simulink model "lab1_3"  (R2026a)
settings: Solver=VariableStepAuto  StopTime=inf
undefined symbols (not defined in the file): Blocking, Non
libraries: amg_usbconverter_n_connect_lib x2
settings Model: Creator=Asus  LastModifiedBy=Asus

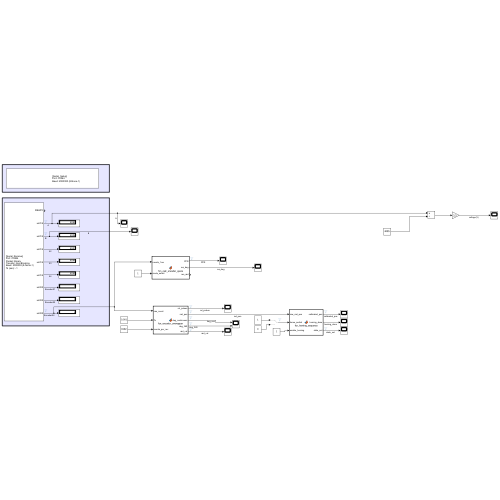
[thumbnail: Simulink's stored preview of the top-level diagram]
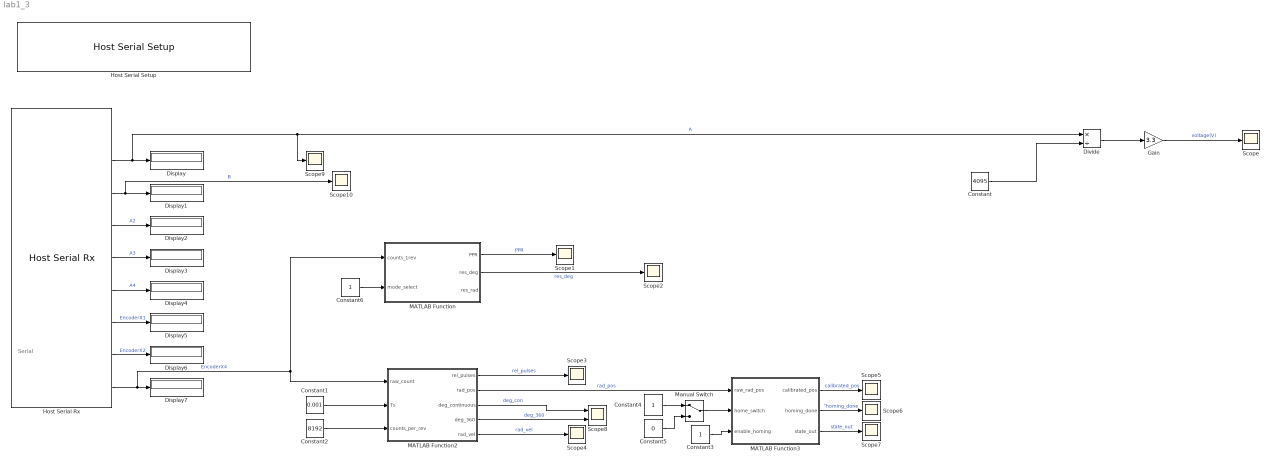
== system lab1_3 ==
  note: Serial
  Constant : Constant  Value=4095
  Constant1 : Constant  Value=0.001
  Constant2 : Constant  Value=8192
  Constant3 : Constant
  Constant4 : Constant  OutDataTypeStr=boolean
  Constant5 : Constant  Value=0  OutDataTypeStr=boolean
  Constant6 : Constant
  Display{,1..7} (8 alike) : Display
  Divide : Product  Inputs=*/
  Gain : Gain  Gain=3.3
  Host Serial Rx : amg_usbconverter_n_connect_lib/Host Serial Rx  conf=rx  port=<auto>  baudrate=2000000  databits=8  parity=None  stopbit=1  flowcontrol=None  transfer=Non-Blocking  timeout=5  packetmode=Binary  enableinitialvalues=off  initialvalues=[]  binheader='25'  binterminator='4E 4E'  porttype_double=0  porttype_single=0  porttype_int8=0  porttype_uint8=0  porttype_int16=0  porttype_uint16=5  porttype_int32=0  porttype_uint32=3  asciiformat='%d,%f'  rx_asciiterminator="CRLF (0x0D 0x0A - \"\\r\\n\")"  tx_asciiterminator="CRLF (0x0D 0x0A - \"\\r\\n\")"  sampletime=0.001  enablecustomportlabel=off  cinputportlabel=0  coutputportlabel=A  portpinstr=0  blockid=HostSerialRx  inputporttype=[]  inputportwidth=[]  inputportlabel={}  outputporttype=[3 5 5 5 5 5 7 7 7]  outputportwidth=[1 1 1 1 1 1 1 1 1]  outputportlabel={'READY','uint16','uint16','uint16','uint16','uint16','uint32','uint32','uint32'}  compat=0  optionstring=[]  autoport='COM4'
  Host Serial Setup : amg_usbconverter_n_connect_lib/Host Serial Setup  conf=setup  port=<auto>  baudrate=2000000  databits=8  parity=None  stopbit=1  flowcontrol=None  transfer=Blocking  timeout=2  packetmode=Binary  initialvalues=[]  binheader='7E 7E'  binterminator='03 03'  porttype_double=0  porttype_single=1  porttype_int8=0  porttype_uint8=0  porttype_int16=0  porttype_uint16=0  porttype_int32=0  porttype_uint32=2  asciiformat='%d %u %x'  rx_asciiterminator="CRLF (0x0D 0x0A - \"\\r\\n\")"  tx_asciiterminator="CRLF (0x0D 0x0A - \"\\r\\n\")"  sampletime=-1  enablecustomportlabel=off  cinputportlabel=0  coutputportlabel=A  portpinstr=0  blockid=HostSerialSetup  inputporttype=[]  inputportwidth=[]  inputportlabel={}  outputporttype=[]  outputportwidth=[]  outputportlabel={}  compat=0  optionstring=[]  autoport='COM4'
  MATLAB Function : MATLAB Function  TreatAsAtomicUnit=on
  MATLAB Function2 : MATLAB Function  TreatAsAtomicUnit=on
  MATLAB Function3 : MATLAB Function  TreatAsAtomicUnit=on
  Manual Switch : ManualSwitch
  Scope{,1..7,9..10} (10 alike) : Scope
      Scope settings: ActiveDisplayYMinimum=-29.471685212947058  ActiveDisplayYMaximum=19.265337201699708
      Scope1 settings: ActiveDisplayYMinimum=-29.471685212947058  ActiveDisplayYMaximum=19.265337201699708
      Scope10 settings: DataLoggingVariableName=ScopeData10
      Scope2 settings: ActiveDisplayYMinimum=-29.471685212947058  ActiveDisplayYMaximum=19.265337201699708  DataLoggingVariableName=ScopeData2
      Scope3 settings: ActiveDisplayYMinimum=-29.471685212947058  ActiveDisplayYMaximum=19.265337201699708  DataLoggingVariableName=ScopeData3
      Scope4 settings: ActiveDisplayYMinimum=-29.471685212947058  ActiveDisplayYMaximum=19.265337201699708  DataLoggingVariableName=ScopeData4
      Scope5 settings: ActiveDisplayYMinimum=-29.471685212947058  ActiveDisplayYMaximum=19.265337201699708  DataLoggingVariableName=ScopeData5
      Scope6 settings: ActiveDisplayYMinimum=-29.471685212947058  ActiveDisplayYMaximum=19.265337201699708  DataLoggingVariableName=ScopeData6
      Scope7 settings: ActiveDisplayYMinimum=-29.471685212947058  ActiveDisplayYMaximum=19.265337201699708  DataLoggingVariableName=ScopeData7
      Scope9 settings: DataLoggingVariableName=ScopeData9
  Scope8 : Scope  NumInputPorts=2
      settings: ActiveDisplayYMinimum=-29.471685212947058  ActiveDisplayYMaximum=19.265337201699708  DataLoggingVariableName=ScopeData8
  wires:
  Host Serial Rx/6 -> Display4/1  "A4"
  Host Serial Rx/9 -> MATLAB Function2/1(raw_count), MATLAB Function/1(counts_1rev), Display7/1  "EncoderX4"
  Constant/1 -> Divide/2
  Host Serial Rx/7 -> Display5/1  "EncoderX1"
  Divide/1 -> Gain/1
  Host Serial Rx/8 -> Display6/1  "EncoderX2"
  Host Serial Rx/3 -> Scope10/1, Display1/1  "B"
  Host Serial Rx/5 -> Display3/1  "A3"
  Host Serial Rx/2 -> Scope9/1, Divide/1, Display/1  "A"
  Gain/1 -> Scope/1  "voltage(V)"
  Host Serial Rx/4 -> Display2/1  "A2"
  Constant1/1 -> MATLAB Function2/2(Ts)
  Constant2/1 -> MATLAB Function2/3(counts_per_rev)
  MATLAB Function2/2(rad_pos) -> MATLAB Function3/1(raw_rad_pos)  "rad_pos"
  Constant3/1 -> MATLAB Function3/3(enable_homing)
  Manual Switch/1 -> MATLAB Function3/2(home_switch)
  Constant4/1 -> Manual Switch/1
  Constant5/1 -> Manual Switch/2
  Constant6/1 -> MATLAB Function/2(mode_select)
  MATLAB Function/1(PPR) -> Scope1/1  "PPR"
  MATLAB Function/2(res_deg) -> Scope2/1  "res_deg"
  MATLAB Function2/5(rad_vel) -> Scope4/1  "rad_vel"
  MATLAB Function2/1(rel_pulses) -> Scope3/1  "rel_pulses"
  MATLAB Function3/1(calibrated_pos) -> Scope5/1  "calibrated_pos"
  MATLAB Function3/2(homing_done) -> Scope6/1  "้homing_done"
  MATLAB Function3/3(state_out) -> Scope7/1  "state_out"
  MATLAB Function2/3(deg_continuous) -> Scope8/1  "deg_con"
  MATLAB Function2/4(deg_360) -> Scope8/2  "deg_360"

== matlab function lab1_3/MATLAB Function ==
  data: counts_1rev input; PPR output; mode_select input; res_deg output; res_rad output
function [PPR, res_deg, res_rad] = fcn_calc_encoder_specs(counts_1rev, mode_select)
% FCN_CALC_ENCODER_SPECS
% คำนวณ PPR และ Angular Resolution (แปลง Type เป็น double ป้องกัน Type Mismatch)

% 1. บังคับแปลง Input ทุกตัวเป็น double ป้องกันการตัดเศษทศนิยมและ Data Type ขัดแย้ง
c = double(counts_1rev);
m = double(mode_select);

% 2. คำนวณค่าตามเงื่อนไข
if c > 0 && m > 0
    PPR     = c / m;
    res_deg = 360.0 / c;
    res_rad = (2.0 * pi) / c;
else
    PPR     = 0.0;
    res_deg = 0.0;
    res_rad = 0.0;
end
end

== matlab function lab1_3/MATLAB Function2 ==
  data: raw_count input; rel_pulses output; Ts input; counts_per_rev input; rad_pos output; deg_continuous output; deg_360 output; rad_vel output
function [rel_pulses, rad_pos, deg_continuous, deg_360, rad_vel] = fcn_encoder_unwrapper(raw_count, Ts, counts_per_rev)
    persistent prev_raw accumulated_pulses prev_rad_pos vel_buffer is_initialized;
    
    MAX_PERIOD = 65536; 
    HALF_PERIOD = MAX_PERIOD / 2;
    WINDOW_SIZE = 15; % ขนาดบัฟเฟอร์เฉลี่ยความเร็ว (ปรับเพิ่มได้ 10 - 25)

    if isempty(is_initialized)
        prev_raw = double(raw_count);
        accumulated_pulses = 0.0;
        prev_rad_pos = 0.0;
        vel_buffer = zeros(1, WINDOW_SIZE);
        is_initialized = true;
    end

    raw_d = double(raw_count);
    ts_d  = double(Ts);
    cpr_d = double(counts_per_rev);

    % 1. Unwrap Logic
    delta_raw = raw_d - prev_raw;
    if delta_raw > HALF_PERIOD
        delta_raw = delta_raw - MAX_PERIOD;
    elseif delta_raw < -HALF_PERIOD
        delta_raw = delta_raw + MAX_PERIOD;
    end

    accumulated_pulses = accumulated_pulses + delta_raw;
    rel_pulses = accumulated_pulses;
    prev_raw = raw_d;

    % 2. ตำแหน่งเชิงมุม
    if cpr_d > 0
        rad_pos = (accumulated_pulses / cpr_d) * (2.0 * pi);
        deg_continuous = (accumulated_pulses / cpr_d) * 360.0;
        deg_360 = mod(deg_continuous, 360.0);
        if deg_360 < 0
            deg_360 = deg_360 + 360.0;
        end
    else
        rad_pos = 0.0;
        deg_continuous = 0.0;
        deg_360 = 0.0;
    end

    % 3. คำนวณความเร็วพร้อม Moving Average Filter
    if ts_d > 0
        raw_vel = (rad_pos - prev_rad_pos) / ts_d;
        % เลื่อนค่าในบัฟเฟอร์และนำค่าใหม่เข้าไปเฉลี่ย
        vel_buffer = [vel_buffer(2:end), raw_vel];
        rad_vel = mean(vel_buffer);
    else
        rad_vel = 0.0;
    end
    
    prev_rad_pos = rad_pos;
end

== matlab function lab1_3/MATLAB Function3 ==
  data: raw_rad_pos input; calibrated_pos output; home_switch input; enable_homing input; homing_done output; state_out output
function [calibrated_pos, homing_done, state_out] = fcn_homing_sequence(raw_rad_pos, home_switch, enable_homing)
% FCN_HOMING_SEQUENCE
% จัดการกระบวนการ Homing เพื่อรีเซ็ตตำแหน่งสัมบูรณ์เริ่มต้นที่ศูนย์
%
% Inputs:
%   raw_rad_pos    : ตำแหน่งมุมเรเดียนจากบล็อก Unwrapper (rad)
%   home_switch    : สถานะสัญญาณสวิตช์ Home (1 = ชนสวิตช์, 0 = ไม่ชน)
%   enable_homing  : คำสั่งเริ่มกระบวนการ Homing (Trigger / Logic 1)
%
% Outputs:
%   calibrated_pos : ตำแหน่งที่เทียบจุด Home แล้ว (rad)
%   homing_done    : สถานะเสร็จสิ้นการ Homing (1 = Done, 0 = Not yet)
%   state_out      : รหัสสถานะปัจจุบัน (0: Idle, 1: Homing, 2: Completed)

    % ตัวแปรเก็บสถานะข้ามรอบ
    persistent state home_offset prev_switch is_init;

    if isempty(is_init)
        state = uint8(0);       % 0: Idle, 1: Searching Home, 2: Completed
        home_offset = 0.0;
        prev_switch = false;
        is_init = true;
    end

    % สลับสถานะตามลำดับ Homing Sequence
    switch state
        case 0 % Idle State
            if enable_homing
                state = uint8(1); % เริ่มเข้าสู่โหมดค้นหา Home
            end
            
        case 1 % Searching / Waiting for Home Trigger
            % ตรวจจับ Rising Edge ของสวิตช์ Home (เมื่อแกนหมุนเข้าสัมผัสสวิตช์)
            if home_switch && ~prev_switch
                home_offset = raw_rad_pos; % บันทึกตำแหน่งจุด Home ไว้เป็น Offset
                state = uint8(2);          % เปลี่ยนสถานะเป็นเสร็จสมบูรณ์
            end
            
        case 2 % Completed State
            if ~enable_homing
                state = uint8(0); % คืนสถานะ Idle เมื่อคำสั่ง Homing ปลดออก
            end
    end

    prev_switch = home_switch;

    % ส่งค่าตำแหน่งที่ชดเชยจุด Home แล้ว
    calibrated_pos = raw_rad_pos - home_offset;
    homing_done = (state == uint8(2));
    state_out = state;
end
